simulink model "practico_3_bumpless"  (R2024b)
settings: Solver=FixedStepAuto  StartTime=0.0  StopTime=700  FixedStep=0.1  RelTol=1e-3
values from neighbouring files (symbols this model uses):
  F_in = 0.0035    [tp3_inicio.m]
  F_out_sin_k = a*sqrt(2*g)    [tp3_inicio.m]
  h_list = [0.2, 0.4, 0.6, 0.8]    [tp3_inicio.m]
  k_list = zeros(1, length(h_list))    [tp3_inicio.m]
  r_0 = 0.05    [tp3_inicio.m]
  theta = 60    [tp3_inicio.m]
undefined symbols (not defined in the file or in its folder): A, B, C, D
libraries: simulink x3, slpidlib x1
settings Model: Creator=trulscarlson  LastModifiedBy=trulscarlson
settings DebuggingCC: UnconnectedInputMsg=warning  UnconnectedOutputMsg=warning  UnconnectedLineMsg=warning
settings ModelReferenceCC: EnableRefExpFcnMdlSchedulingChecks=on
settings RTWCC: GPUComputeCapability=3.5  DLArmComputeVersion=19.05

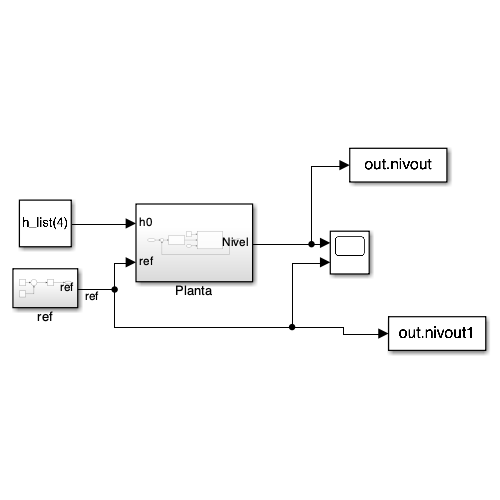
[thumbnail: Simulink's stored preview of the top-level diagram]
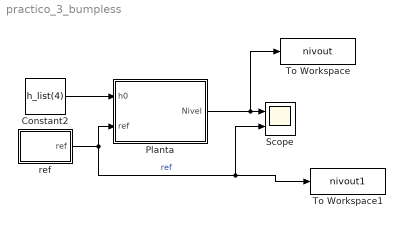
== system practico_3_bumpless ==
  Constant2 : Constant  Value=h_list(4)
  Planta : Subsystem
  Scope : Scope  NumInputPorts=2
  To Workspace : ToWorkspace  VariableName=nivout  SaveFormat=Timeseries  SampleTime=-1
  To Workspace1 : ToWorkspace  VariableName=nivout1  SaveFormat=Timeseries  SampleTime=-1
  ref : Subsystem
  wires:
  Planta/1(Nivel) -> To Workspace/1, Scope/1
  Constant2/1 -> Planta/1(h0)
  ref/1(ref) -> Planta/2(ref), To Workspace1/1, Scope/2  "ref"

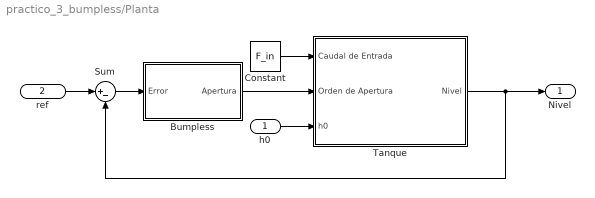
== system practico_3_bumpless/Planta ==
  h0 : Inport
  ref : Inport  Port=2
  Bumpless : Subsystem
  Constant : Constant  Value=F_in
  Sum : Sum  Inputs=|+-
  Tanque : Subsystem
  Nivel : Outport
  wires:
  h0/1 -> Tanque/3(h0)
  Constant/1 -> Tanque/1(Caudal de Entrada)
  Tanque/1(Nivel) -> Sum/2, Nivel/1
  ref/1 -> Sum/1
  Bumpless/1(Apertura) -> Tanque/2(Orden de Apertura)
  Sum/1 -> Bumpless/1(Error)

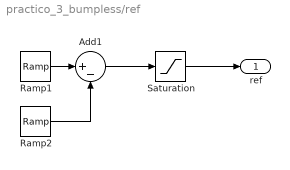
== system practico_3_bumpless/ref ==
  Add1 : Sum  Inputs=|+-
  Ramp1 : simulink/Sources/Ramp  slope=0.00400  start=250  InitialOutput=h_list(1)
  Ramp2 : simulink/Sources/Ramp  slope=0.00400  start=450  InitialOutput=0
  Saturation : Saturate  UpperLimit=h_list(4)  LowerLimit=h_list(1)
  ref : Outport  VectorParamsAs1DForOutWhenUnconnected=off
  wires:
  Ramp2/1 -> Add1/2
  Ramp1/1 -> Add1/1
  Add1/1 -> Saturation/1
  Saturation/1 -> ref/1

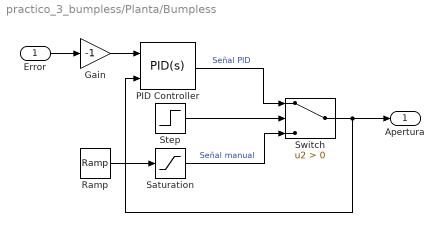
== system practico_3_bumpless/Planta/Bumpless ==
  Error : Inport
  Gain : Gain  Gain=-1
  PID Controller : slpidlib/PID Controller  Controller=PID  Form=Parallel  TimeDomain=Continuous-time  UseExternalTs=off  SampleTime=-1  IntegratorMethod=Forward Euler  FilterMethod=Forward Euler  ControllerParametersSource=internal  P=15.33  I=0.38  UseKiTs=off  D=119.13  UseExternalDerivativeSource=off  N=10  UseFilter=on  TunerSelectOption=Transfer Function Based (PID Tuner App)  InitialConditionSource=internal  InitialConditionForIntegrator=k_list(4)  InitialConditionForFilter=0  DifferentiatorICPrevScaledInput=0  ExternalReset=none  TrackingMode=on  Kt=1  LimitOutput=on  SatLimitsSource=internal  UpperSaturationLimit=1  LowerSaturationLimit=0  LinearizeAsGain=on  AntiWindupMode=clamping  Kb=1  LimitIntegrator=off  UpperIntegratorSaturationLimit=inf  LowerIntegratorSaturationLimit=-inf  POutMin=[]  POutMax=[]  IOutMin=[]  IOutMax=[]  DOutMin=[]  DOutMax=[]  NOutMin=[]  NOutMax=[]  SumOutMin=[]  SumOutMax=[]  SaturationOutMin=[]  SaturationOutMax=[]  PParamMin=[]  PParamMax=[]  IParamMin=[]  IParamMax=[]  DParamMin=[]  DParamMax=[]  NParamMin=[]  NParamMax=[]  KbParamMin=[]  KbParamMax=[]  KtParamMin=[]  KtParamMax=[]  KbOutMin=[]  KbOutMax=[]  KtOutMin=[]  KtOutMax=[]  IntegratorOutMin=[]  IntegratorOutMax=[]  FilterOutMin=[]  FilterOutMax=[]  SumI1OutMin=[]  SumI1OutMax=[]  SumI2OutMin=[]  SumI2OutMax=[]  SumI3OutMin=[]  SumI3OutMax=[]  SumI4OutMin=[]  SumI4OutMax=[]  SumDOutMin=[]  SumDOutMax=[]  DifferentiatorOutMin=[]  DifferentiatorOutMax=[]  FilterDiffOutCoefMin=[]  FilterDiffOutCoefMax=[]  ReciprocalOutMin=[]  ReciprocalOutMax=[]  SumDenOutMin=[]  SumDenOutMax=[]  SumNumOutMin=[]  SumNumOutMax=[]  DivideOutMin=[]  DivideOutMax=[]  UdiffTsProdOutMin=[]  UdiffTsProdOutMax=[]  NTsProdOutMin=[]  NTsProdOutMax=[]  UintegralTsProdOutMin=[]  UintegralTsProdOutMax=[]  UngainTsProdOutMin=[]  UngainTsProdOutMax=[]  ClampingZeroOutDataTypeStr=Inherit: Inherit via back propagation  ClampingZeroOutMin=[]  ClampingZeroOutMax=[]  FilterDenConstantOutDataTypeStr=Inherit: Inherit via back propagation  FilterDenConstantOutMin=[]  FilterDenConstantOutMax=[]  PCopyOutDataTypeStr=Inherit: Inherit via back propagation  PCopyOutMin=[]  PCopyOutMax=[]  NCopyOutDataTypeStr=Inherit: Inherit via back propagation  NCopyOutMin=[]  NCopyOutMax=[]  IntegratorContinuousStateAttributes=''  IntegratorStateMustResolveToSignalObject=off  IntegratorRTWStateStorageClass=Auto  FilterContinuousStateAttributes=''  FilterStateMustResolveToSignalObject=off  FilterRTWStateStorageClass=Auto  ParallelPVariant=InternalParameters  IdealPVariant=Disabled  IVariant=InternalParameters  DVariant=InternalParameters  IntegratorVariant=Continuous  SatVariant=Enabled  AWVariant=ContClampingParallel  PCopyVariant=Disabled  TRVariant=Enabled  FdbkBlocksVariant=Forward  IdealPFdbkVariant=Disabled  SatFdbkVariant=Disabled  DerivativeFilterVariant=ContFilter  NVariant=InternalParameters  NCopyVariant=Disabled  FilterICVariant=InternalICsFilter  IntegratorICVariant=InternalICs  ExternalResetVariant=Disabled  TRSumVariant=TrackingMode  SumFdbkVariant=Disabled  SumVariant=Sum_PID  TsampFilterVariant=InternalTs  TsampNgainVariant=Passthrough  TsampIntegralVariant=Disabled_SignalSpec  ExternalSaturationOutDataTypeStr=Inherit: Same as second input  DerivativeSourceVariant=ErrorSignal  PreIntVariant=InternalPreInt
  Ramp : simulink/Sources/Ramp  slope=0.05  start=0  InitialOutput=k_list(4)
  Saturation : Saturate  UpperLimit=k_list(1)  LowerLimit=0
  Step : Step  Time=220  SampleTime=0
  Switch : Switch  Criteria=u2 > Threshold  SaturateOnIntegerOverflow=off  InputSameDT=off
  Apertura : Outport
  wires:
  Switch/1 -> PID Controller/2, Apertura/1
  Step/1 -> Switch/2
  Ramp/1 -> Saturation/1
  Saturation/1 -> Switch/3  "Señal manual"
  Gain/1 -> PID Controller/1
  Error/1 -> Gain/1
  PID Controller/1 -> Switch/1  "Señal PID"

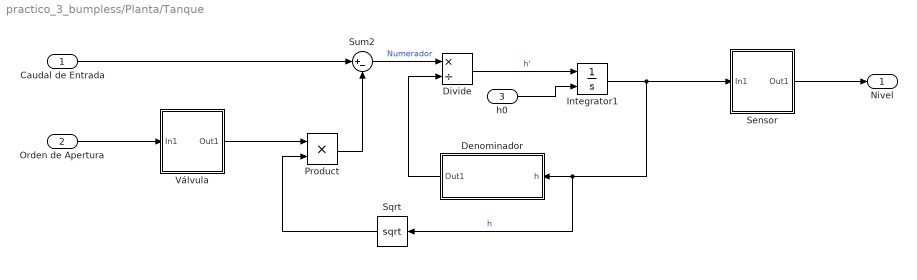
== system practico_3_bumpless/Planta/Tanque ==
  Caudal de Entrada : Inport
  Orden de Apertura : Inport  Port=2
  h0 : Inport  Port=3
  Denominador : Subsystem
  Divide : Product  Inputs=*/
  Integrator1 : Integrator  InitialConditionSource=external  InitialCondition=h_list(5)
  Product : Product
  Sensor : Subsystem
  Sqrt : Sqrt
  Sum2 : Sum  Inputs=|+-
  Válvula : Subsystem
  Nivel : Outport
  wires:
  Product/1 -> Sum2/2
  Divide/1 -> Integrator1/1  "h'"
  Denominador/1(Out1) -> Divide/2
  Integrator1/1 -> Sensor/1(In1), Sqrt/1, Denominador/1(h)  "h"
  Sum2/1 -> Divide/1  "Numerador"
  Sqrt/1 -> Product/2
  Caudal de Entrada/1 -> Sum2/1
  Orden de Apertura/1 -> Válvula/1(In1)
  Válvula/1(Out1) -> Product/1
  h0/1 -> Integrator1/2
  Sensor/1(Out1) -> Nivel/1

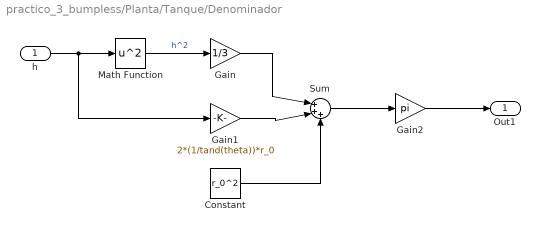
== system practico_3_bumpless/Planta/Tanque/Denominador ==
  h : Inport
  Constant : Constant  Value=r_0^2
  Gain : Gain  Gain=1/3
  Gain1 : Gain  Gain=2*(1/tand(theta))*r_0
  Gain2 : Gain  Gain=pi
  Math Function : Math  Operator=square
  Sum : Sum  Inputs=|+++
  Out1 : Outport
  wires:
  h/1 -> Gain1/1, Math Function/1
  Math Function/1 -> Gain/1  "h^2"
  Gain/1 -> Sum/1
  Gain1/1 -> Sum/2
  Constant/1 -> Sum/3
  Sum/1 -> Gain2/1
  Gain2/1 -> Out1/1

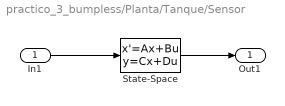
== system practico_3_bumpless/Planta/Tanque/Sensor ==
  In1 : Inport
  State-Space : StateSpace  A=A  B=B  C=C  D=D  InitialCondition=h_list(4)*10
  Out1 : Outport
  wires:
  In1/1 -> State-Space/1
  State-Space/1 -> Out1/1

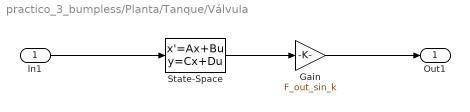
== system practico_3_bumpless/Planta/Tanque/Válvula ==
  In1 : Inport
  Gain : Gain  Gain=F_out_sin_k
  State-Space : StateSpace  A=A  B=B  C=C  D=D  InitialCondition=k_list(4)*10
  Out1 : Outport
  wires:
  State-Space/1 -> Gain/1
  Gain/1 -> Out1/1
  In1/1 -> State-Space/1
